simulink subsystem "COMP_QUAD_COL_SYS"  (R2025b)
settings: Solver=VariableStepAuto  StartTime=0.0  StopTime=10.0  RelTol=1e-3
libraries: sm_lib x8
settings Model: Creator=bhorton  LastModifiedBy=bhorton

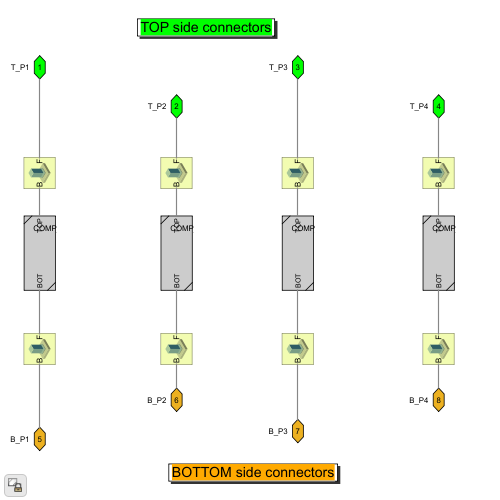
[thumbnail: Simulink's stored preview of the top-level diagram]
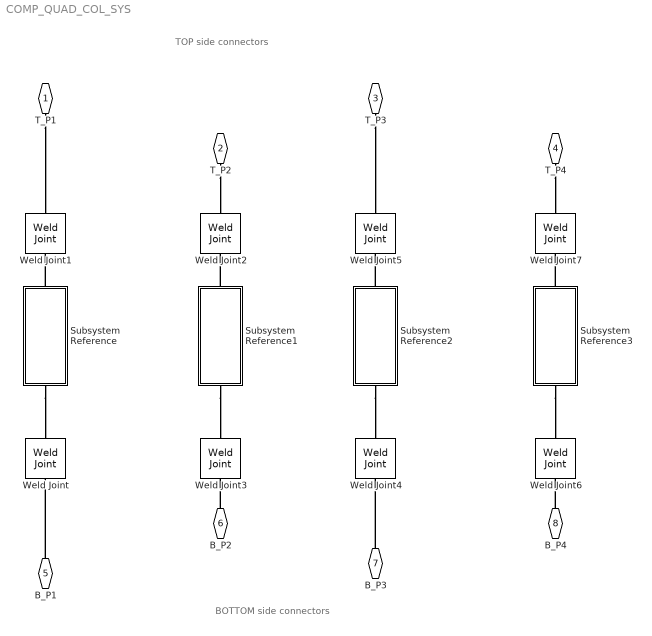
== system COMP_QUAD_COL_SYS ==
  note: TOP side connectors
  note: BOTTOM side connectors
  Subsystem Reference{,1..3} (4 alike) : Subsystem  ReferencedSubsystem=COMP_COL_SYS
  Weld Joint{,1..7} (8 alike) : sm_lib/Joints/Weld Joint  JointMode=Normal  CompositeWrenchDir=FollowerOnBase  CompositeWrenchFrame=BaseFrame  SenseConstraintForce=off  SenseConstraintTorque=off  SenseTotalForce=off  SenseTotalTorque=off
  T_P1 : PMIOPort  Side=Left
  T_P2 : PMIOPort  Port=2  Side=Left
  T_P3 : PMIOPort  Port=3  Side=Left
  T_P4 : PMIOPort  Port=4  Side=Left
  B_P1 : PMIOPort  Port=5  Side=Right
  B_P2 : PMIOPort  Port=6  Side=Right
  B_P3 : PMIOPort  Port=7  Side=Right
  B_P4 : PMIOPort  Port=8  Side=Right
  connections:
  T_P2/RConn1 -- Weld Joint2/RConn1
  Subsystem Reference/RConn1 -- Weld Joint/RConn1
  Subsystem Reference2/LConn1 -- Weld Joint5/LConn1
  B_P4/RConn1 -- Weld Joint6/LConn1
  T_P3/RConn1 -- Weld Joint5/RConn1
  T_P1/RConn1 -- Weld Joint1/RConn1
  Subsystem Reference1/LConn1 -- Weld Joint2/LConn1
  B_P3/RConn1 -- Weld Joint4/LConn1
  Subsystem Reference3/RConn1 -- Weld Joint6/RConn1
  Subsystem Reference2/RConn1 -- Weld Joint4/RConn1
  T_P4/RConn1 -- Weld Joint7/RConn1
  Subsystem Reference1/RConn1 -- Weld Joint3/RConn1
  B_P1/RConn1 -- Weld Joint/LConn1
  Subsystem Reference3/LConn1 -- Weld Joint7/LConn1
  B_P2/RConn1 -- Weld Joint3/LConn1
  Subsystem Reference/LConn1 -- Weld Joint1/LConn1
